simulink model "ABS_RCAC_ESC_Juan"  (R2023a)
settings: Solver=FixedStepDiscrete  StartTime=0.0  StopTime=100000  FixedStep=1  RelTol=1e-3
undefined symbols (not defined in the file or in its folder): B, DiscIntNeverNeededParam, I, lambda_zero, m, R, u_asterix
settings Model: Creator=PhDstudent1  LastModifiedBy=PhDstudent1
settings DataIOCC: ReturnWorkspaceOutputsName=out4

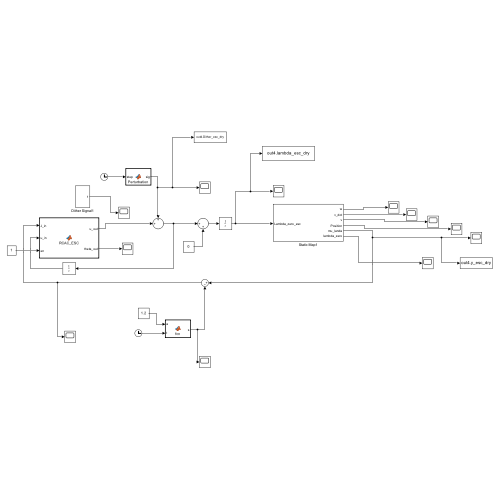
[thumbnail: Simulink's stored preview of the top-level diagram]
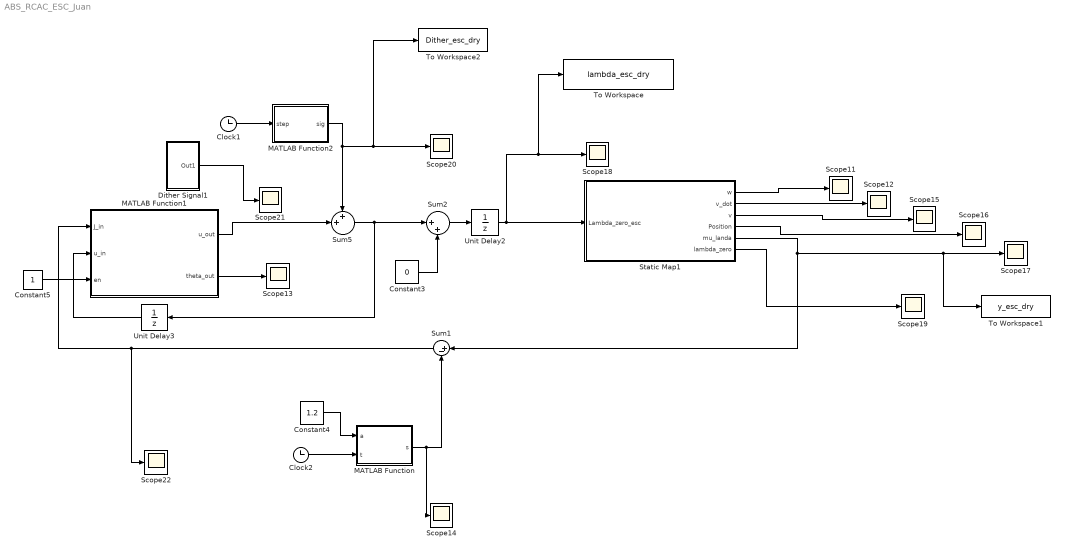
== system ABS_RCAC_ESC_Juan ==
  Clock1 : Clock
  Clock2 : Clock
  Constant3 : Constant  Value=0
  Constant4 : Constant  Value=1.2
  Constant5 : Constant
  Dither Signal1 : Subsystem
  MATLAB Function : MATLAB Function  TreatAsAtomicUnit=on
  MATLAB Function1 : MATLAB Function  TreatAsAtomicUnit=on
  MATLAB Function2 : MATLAB Function  TreatAsAtomicUnit=on
  Scope{11..22} (12 alike) : Scope
  Static Map1 : Subsystem
  Sum1 : Sum  Inputs=|+-
  Sum2 : Sum  Inputs=|++
  Sum5 : Sum  Inputs=++|
  To Workspace : ToWorkspace  VariableName=lambda_esc_dry  SaveFormat=Timeseries  SampleTime=-1
  To Workspace1 : ToWorkspace  VariableName=y_esc_dry  SaveFormat=Timeseries  SampleTime=-1
  To Workspace2 : ToWorkspace  VariableName=Dither_esc_dry  SaveFormat=Timeseries  SampleTime=-1
  Unit Delay2 : UnitDelay  InitialCondition=0.3  SampleTime=-1  HasFrameUpgradeWarning=on
  Unit Delay3 : UnitDelay  SampleTime=-1  HasFrameUpgradeWarning=on
  wires:
  Static Map1/3(v) -> Scope15/1
  Sum2/1 -> Unit Delay2/1
  MATLAB Function/1(s) -> Sum1/2, Scope14/1
  Clock2/1 -> MATLAB Function/2(t)
  Constant5/1 -> MATLAB Function1/3(en)
  Static Map1/5(mu_landa) -> Sum1/1, To Workspace1/1, Scope17/1
  Constant3/1 -> Sum2/2
  Clock1/1 -> MATLAB Function2/1(step)
  Sum1/1 -> MATLAB Function1/1(J_in), Scope22/1
  Constant4/1 -> MATLAB Function/1(a)
  Unit Delay3/1 -> MATLAB Function1/2(u_in)
  MATLAB Function2/1(sig) -> Sum5/1, To Workspace2/1, Scope20/1
  Static Map1/4(Position) -> Scope16/1
  Dither Signal1/1(Out1) -> Scope21/1
  Static Map1/2(v_dot) -> Scope12/1
  Static Map1/6(lambda_zero) -> Scope19/1
  MATLAB Function1/2(theta_out) -> Scope13/1
  Sum5/1 -> Unit Delay3/1, Sum2/1
  MATLAB Function1/1(u_out) -> Sum5/2
  Unit Delay2/1 -> Static Map1/1(Lambda_zero_esc), To Workspace/1, Scope18/1
  Static Map1/1(w) -> Scope11/1

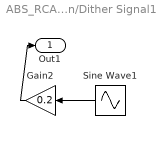
== system ABS_RCAC_ESC_Juan/Dither Signal1 ==
  Gain2 : Gain  Gain=0.2
  Sine Wave1 : Sin  Frequency=30  SampleTime=0
  Out1 : Outport
  wires:
  Sine Wave1/1 -> Gain2/1
  Gain2/1 -> Out1/1

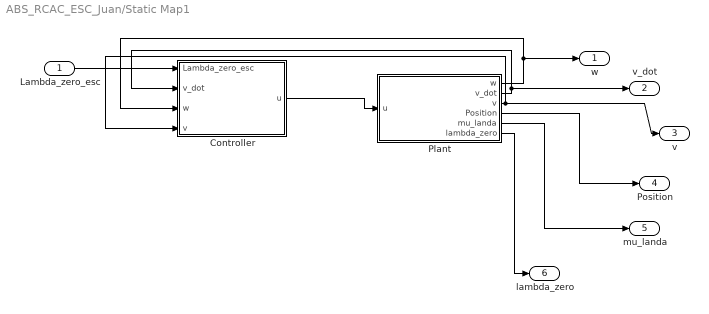
== system ABS_RCAC_ESC_Juan/Static Map1 ==
  Lambda_zero_esc : Inport
  Controller : Subsystem
  Plant : Subsystem
  w : Outport
  v_dot : Outport  Port=2
  v : Outport  Port=3
  Position : Outport  Port=4
  mu_landa : Outport  Port=5
  lambda_zero : Outport  Port=6
  wires:
  Controller/1(u) -> Plant/1(u)
  Plant/2(v_dot) -> v_dot/1, Controller/2(v_dot)
  Plant/3(v) -> Controller/4(v), v/1
  Lambda_zero_esc/1 -> Controller/1(Lambda_zero_esc)
  Plant/1(w) -> w/1, Controller/3(w)
  Plant/5(mu_landa) -> mu_landa/1
  Plant/4(Position) -> Position/1
  Plant/6(lambda_zero) -> lambda_zero/1

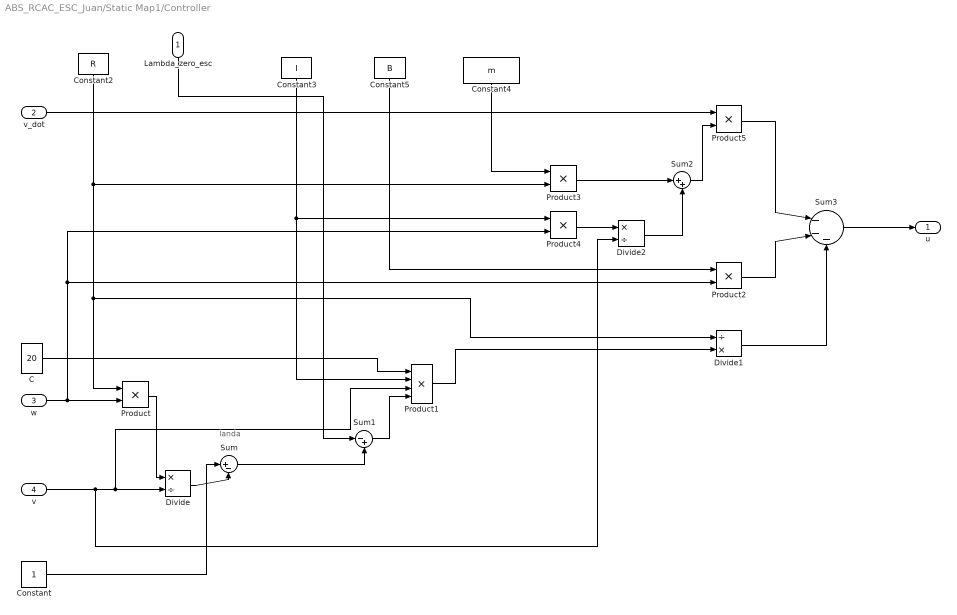
== system ABS_RCAC_ESC_Juan/Static Map1/Controller ==
  note: landa
  Lambda_zero_esc : Inport
  v_dot : Inport  Port=2
  w : Inport  Port=3
  v : Inport  Port=4
  C : Constant  Value=20
  Constant : Constant
  Constant2 : Constant  Value=R
  Constant3 : Constant  Value=I
  Constant4 : Constant  Value=m
  Constant5 : Constant  Value=B
  Divide : Product  Inputs=*/
  Divide1 : Product  Inputs=/*
  Divide2 : Product  Inputs=*/
  Product{,2..5} (5 alike) : Product
  Product1 : Product  Inputs=4
  Sum : Sum  Inputs=|+-
  Sum1 : Sum  Inputs=|-+
  Sum2 : Sum  Inputs=|++
  Sum3 : Sum  Inputs=|---
  u : Outport
  wires:
  Constant/1 -> Sum/1
  v/1 -> Divide2/2, Product1/3, Divide/2
  Divide/1 -> Sum/2
  w/1 -> Product4/2, Product2/2, Product/2
  Constant2/1 -> Product3/2, Product/1, Divide1/1
  Product/1 -> Divide/1
  Sum/1 -> Sum1/2
  Lambda_zero_esc/1 -> Sum1/1
  Sum1/1 -> Product1/4
  Constant3/1 -> Product1/2, Product4/1
  C/1 -> Product1/1
  Product1/1 -> Divide1/2
  Constant5/1 -> Product2/1
  Constant4/1 -> Product3/1
  Product4/1 -> Divide2/1
  Product3/1 -> Sum2/1
  Divide2/1 -> Sum2/2
  Sum2/1 -> Product5/2
  v_dot/1 -> Product5/1
  Product5/1 -> Sum3/1
  Product2/1 -> Sum3/2
  Divide1/1 -> Sum3/3
  Sum3/1 -> u/1

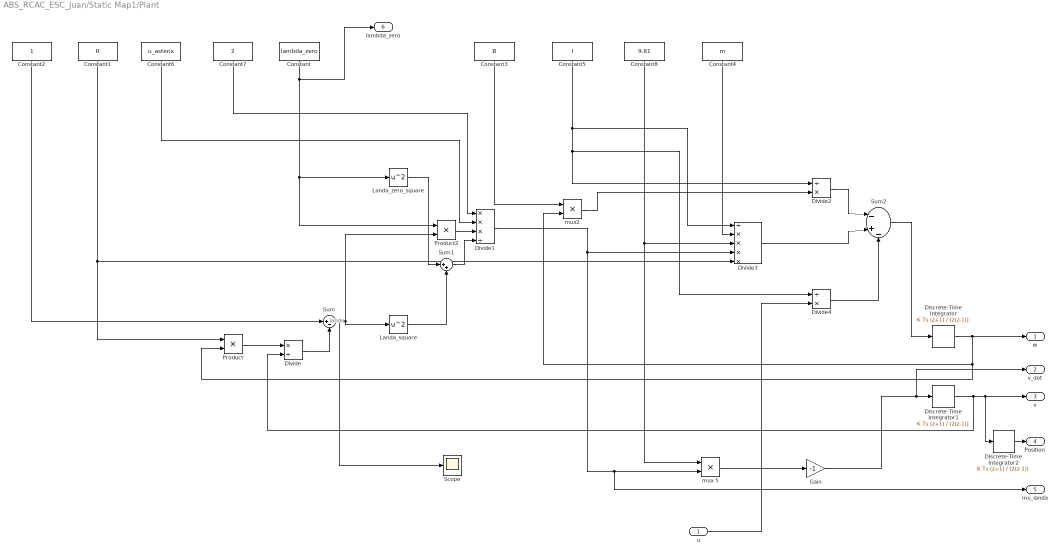
== system ABS_RCAC_ESC_Juan/Static Map1/Plant ==
  note: landa
  u : Inport
  Constant : Constant  Value=lambda_zero
  Constant1 : Constant  Value=R
  Constant2 : Constant
  Constant3 : Constant  Value=B
  Constant4 : Constant  Value=m
  Constant5 : Constant  Value=I
  Constant6 : Constant  Value=u_asterix
  Constant7 : Constant  Value=2
  Constant8 : Constant  Value=9.81
  Discrete-Time Integrator : DiscreteIntegrator  IntegratorMethod=Integration: Trapezoidal  InitialCondition=121.212  SampleTime=-1  ICPrevOutput=DiscIntNeverNeededParam  ICPrevScaledInput=DiscIntNeverNeededParam
  Discrete-Time Integrator1 : DiscreteIntegrator  IntegratorMethod=Integration: Trapezoidal  InitialCondition=1200/36  SampleTime=-1  ICPrevOutput=DiscIntNeverNeededParam  ICPrevScaledInput=DiscIntNeverNeededParam
  Discrete-Time Integrator2 : DiscreteIntegrator  IntegratorMethod=Integration: Trapezoidal  SampleTime=-1  ICPrevOutput=DiscIntNeverNeededParam  ICPrevScaledInput=DiscIntNeverNeededParam
  Divide : Product  Inputs=*/
  Divide1 : Product  Inputs=***/
  Divide2 : Product  Inputs=/*
  Divide3 : Product  Inputs=/****
  Divide4 : Product  Inputs=/*
  Gain : Gain  Gain=-1
  "Landa_square " : Math  Operator=square  SignedPower=on
  "Landa_zero_square " : Math  Operator=square  SignedPower=on
  Product : Product
  Product2 : Product
  Scope : Scope
  Sum : Sum  Inputs=|+-
  Sum1 : Sum  Inputs=|++
  Sum2 : Sum  Inputs=|-+-
  mux 5 : Product
  mux2 : Product
  w : Outport
  v_dot : Outport  Port=2
  v : Outport  Port=3
  Position : Outport  Port=4
  mu_landa : Outport  Port=5
  lambda_zero : Outport  Port=6
  wires:
  Constant1/1 -> Product/1, Divide3/5
  Discrete-Time Integrator/1 -> mux2/2, Product/2, w/1
  Product/1 -> Divide/1
  Discrete-Time Integrator1/1 -> Divide/2, Discrete-Time Integrator2/1, v/1
  Constant2/1 -> Sum/1
  Divide/1 -> Sum/2
  Constant7/1 -> Divide1/1
  Constant6/1 -> Divide1/2
  Constant/1 -> lambda_zero/1, "Landa_zero_square "/1, Product2/1
  Sum/1 -> Scope/1, Product2/2, "Landa_square "/1
  "Landa_zero_square "/1 -> Sum1/1
  "Landa_square "/1 -> Sum1/2
  Product2/1 -> Divide1/3
  Sum1/1 -> Divide1/4
  Constant3/1 -> mux2/1
  mux2/1 -> Divide2/2
  Constant5/1 -> Divide3/1, Divide4/1, Divide2/1
  Constant4/1 -> Divide3/2
  Constant8/1 -> mux 5/1, Divide3/3
  Divide1/1 -> mu_landa/1, mux 5/2, Divide3/4
  u/1 -> Divide4/2
  Divide2/1 -> Sum2/1
  Divide3/1 -> Sum2/2
  Divide4/1 -> Sum2/3
  Sum2/1 -> Discrete-Time Integrator/1
  mux 5/1 -> Gain/1
  Gain/1 -> Discrete-Time Integrator1/1, v_dot/1
  Discrete-Time Integrator2/1 -> Position/1

== matlab function ABS_RCAC_ESC_Juan/MATLAB Function ==
  data: a input; s output; t input
function s = fcn(a,t)

s = a*exp(0*t);
end

== matlab function ABS_RCAC_ESC_Juan/MATLAB Function1 ==
  settings: updateMethod=DISCRETE  sampleTime=1
  data: J_in input size=1; u_out output size=1; u_in input size=1; en input size=1; theta_out output size=20; Nc parameter size=1
function [u_out, theta_out] = RCAC_ESC(J_in, u_in, en, Nc)

persistent Grad_Est DDRCAC_Cont uouttemp thetaouttemp opts

if isempty(uouttemp)
    opts = RCAC_ESC_KF_SISO_define_opts();
    Grad_Est = grad_est_KF(opts.lu, opts.lz, opts.indi, opts.P0_G, opts.Q, opts.R);
    DDRCAC_Cont = DDRCAC(opts.lu, opts.lz, opts.Nc, opts.P0_C, opts.Ru, opts.nu);
    uouttemp = 0.0;
    thetaouttemp = zeros(2*Nc,1); 
end

theta_out = zeros(20,1); %Due to Max number for Nc = 10, can adjust by changing theta_out size

if en > 0.1
    %% Gradient estimation
    [Grad_Est, grad] = Grad_Est.oneStep(u_in, J_in, en);
    
    %% Gradient to Nf (SISO)
    gradNorm = abs(grad);
    gradNorm(gradNorm<=opts.epsi) = opts.epsi;
    Nf = grad./gradNorm;
    
    %% RCAC with Nf (DDRCAC)
    [DDRCAC_Cont, uouttemp, thetaouttemp] = DDRCAC_Cont.oneStep(u_in, J_in, Nf, 0);

end

u_out = uouttemp(1,1);
% theta_out(1:2*Nc,1) = thetaouttemp(1:2*Nc,1);

end

== matlab function ABS_RCAC_ESC_Juan/MATLAB Function2 ==
  settings: updateMethod=DISCRETE
  data: step input size=1; sig output size=1
function sig = Perturbation(step)
    sig = PertFcnSISO(step);
end
